simulink model "Observable"  (Simulink 8.8)
settings: Solver=VariableStepAuto  StartTime=0.0  StopTime=10.0  RelTol=1e-3
settings Model: Creator=Bonner  LastModifiedBy=Bonner
settings DataIOCC: LimitDataPoints=off  SaveFormat=Dataset  SignalLoggingSaveFormat=Dataset
settings OptimizationCC: LifeSpan=auto
settings DebuggingCC: UnderspecifiedInitializationDetection=Simplified  MergeDetectMultiDrivingBlocksExec=error  FcnCallInpInsideContextMsg=error  StateNameClashWarn=none  SFUnexpectedBacktrackingDiag=error  SFNoUnconditionalDefaultTransitionDiag=error  SFExecutionAtInitializationDiag=warning
settings HardwareCC: ProdBitPerPointer=64  ProdBitPerSizeT=64  ProdBitPerPtrDiffT=64  ProdLargestAtomicFloat=Float  ProdIntDivRoundTo=Zero  ProdEndianess=LittleEndian  ProdWordSize=64  ProdHWDeviceType=Intel->x86-64 (Windows64)
settings ModelReferenceCC: PropagateSignalLabelsOutOfModel=on
settings GRTTargetCC: TargetLangStandard=C99 (ISO)  GeneratePreprocessorConditionals=Use local settings  CombineOutputUpdateFcns=on  GRTInterface=off
settings ConfigComp: CovMetricSettings=dwe  CovHtmlReporting=off  CovSaveCumulativeToWorkspaceVar=off  CovSaveSingleToWorkspaceVar=off  CovExternalEMLEnable=on

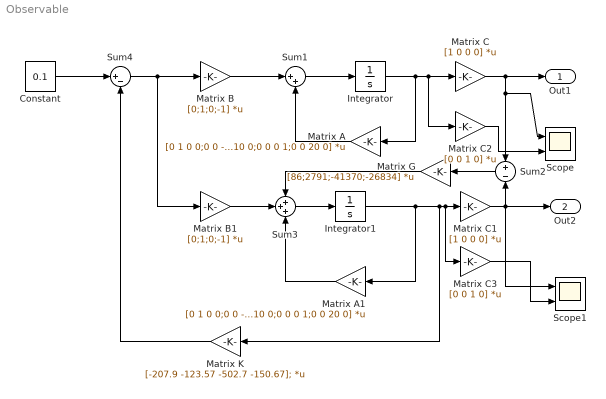
== system Observable ==
  Constant : Constant  Value=0.1
  Integrator : Integrator  InitialCondition=[0 0 0.1 0]
  Integrator1 : Integrator  InitialCondition=[0 0 0.1 0]  AbsoluteTolerance=0.001
  Matrix A : Gain  Gain=[0 1 0 0;0 0 -10 0;0 0 0 1;0 0 20 0]  Multiplication=Matrix(K*u)
  Matrix A1 : Gain  Gain=[0 1 0 0;0 0 -10 0;0 0 0 1;0 0 20 0]  Multiplication=Matrix(K*u)
  Matrix B : Gain  Gain=[0;1;0;-1]  Multiplication=Matrix(K*u)
  Matrix B1 : Gain  Gain=[0;1;0;-1]  Multiplication=Matrix(K*u)
  Matrix C : Gain  Gain=[1 0 0 0]  Multiplication=Matrix(K*u)
  Matrix C1 : Gain  Gain=[1 0 0 0]  Multiplication=Matrix(K*u)
  Matrix C2 : Gain  Gain=[0 0 1 0]  Multiplication=Matrix(K*u)
  Matrix C3 : Gain  Gain=[0 0 1 0]  Multiplication=Matrix(K*u)
  Matrix G : Gain  Gain=[86;2791;-41370;-26834]  Multiplication=Matrix(K*u)
  Matrix K : Gain  Gain=[-207.9 -123.57 -502.7 -150.67];  Multiplication=Matrix(K*u)
  Scope : Scope  NumInputPorts=2
  Scope1 : Scope  NumInputPorts=2
  Sum1 : Sum  Inputs=|++
  Sum2 : Sum  Inputs=+-
  Sum3 : Sum  Inputs=+++
  Sum4 : Sum  Inputs=|+-
  Out1 : Outport
  Out2 : Outport  Port=2
  wires:
  Constant/1 -> Sum4/1
  Matrix B/1 -> Sum1/1
  Sum1/1 -> Integrator/1
  Integrator/1 -> Matrix A/1, Matrix C2/1, Matrix C/1
  Matrix C/1 -> Sum2/1, Scope/1, Out1/1
  Matrix A/1 -> Sum1/2
  Matrix B1/1 -> Sum3/2
  Matrix G/1 -> Sum3/1
  Sum3/1 -> Integrator1/1
  Sum2/1 -> Matrix G/1
  Integrator1/1 -> Matrix A1/1, Matrix K/1, Matrix C3/1, Matrix C1/1
  Matrix C1/1 -> Scope1/1, Out2/1, Sum2/2
  Matrix A1/1 -> Sum3/3
  Matrix K/1 -> Sum4/2
  Sum4/1 -> Matrix B/1, Matrix B1/1
  Matrix C2/1 -> Scope/2
  Matrix C3/1 -> Scope1/2
